simulink model "figure_1_8"  (R2026a)
settings: Solver=ode5  FixedStep=1e-4
settings Model: Creator=yagmu  LastModifiedBy=yagmu

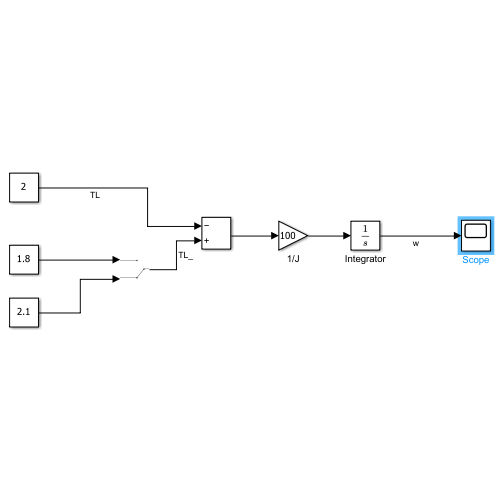
[thumbnail: Simulink's stored preview of the top-level diagram]
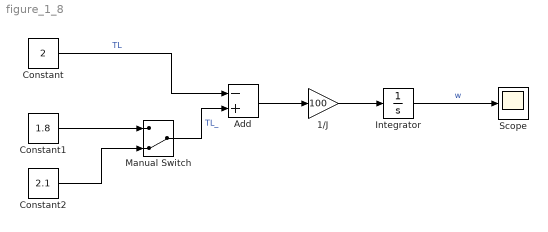
== system figure_1_8 ==
  1/J : Gain  Gain=100
  Add : Sum  Inputs=-+
  Constant : Constant  Value=2
  Constant1 : Constant  Value=1.8
  Constant2 : Constant  Value=2.1
  Integrator : Integrator  InitialCondition=50
  Manual Switch : ManualSwitch  CurrentSetting=0
  Scope : Scope
      settings: ActiveDisplayYMinimum=-59.186536753681821  ActiveDisplayYMaximum=39.630117780702946
  wires:
  Constant/1 -> Add/1  "TL"
  Add/1 -> 1/J/1
  1/J/1 -> Integrator/1
  Integrator/1 -> Scope/1  "w"
  Constant1/1 -> Manual Switch/1
  Constant2/1 -> Manual Switch/2
  Manual Switch/1 -> Add/2  "TL_"
